simulink model "Parent"  (R2024a)
settings: Solver=FixedStepAuto  StartTime=0.0  StopTime=inf  RelTol=1e-3
libraries: androidcommunicationlib x3, androiduilib x3, androidaudiovideolib x2
settings Model: Creator=tamiz  LastModifiedBy=Shesh
settings OptimizationCC: EnhancedBackFolding=on  PassReuseOutputArgsAs=Individual arguments  ZeroExternalMemoryAtStartup=off  ZeroInternalMemoryAtStartup=off  MaxStackSize=64  OptimizeBlockOrder=speed  DifferentSizesBufferReuse=on  OptimizationCustomize=off  EfficientTunableParamExpr=on
settings DebuggingCC: ParameterTunabilityLossMsg=error
settings HardwareCC: ProdBitPerPointer=32  ProdBitPerSizeT=32  ProdBitPerPtrDiffT=32  ProdLargestAtomicInteger=Long  ProdLargestAtomicFloat=Double  ProdWordSize=32  ProdHWDeviceType=ARM Compatible->ARM Cortex  UseEmbeddedCoderFeatures=off  UseSimulinkCoderFeatures=off
settings SFSimCC: MATLABDynamicMemAlloc=off
settings RTWCC: Description=Embedded Coder  SystemTargetFile=ert.tlc  HardwareBoard=Android Device  TLCOptions="-aInlineSetEventsForThisBaseRateFcn=TLC_FALSE -aSuppressMultiTaskScheduler=TLC_FALSE  -aRateBasedStepFcn=0"  TemplateMakefile=ert_default_tmf  RTWVerbose=off  Toolchain=Android SDK/NDK Tools  GPUComputeCapability=3.5
settings CodeAppCC: ForceParamTrailComments=on  IgnoreCustomStorageClasses=off  OperatorAnnotations=on  SimulinkDataObjDesc=on  SFDataObjDesc=on  InsertBlockDesc=on
settings ERTTargetCC: SupportNonInlinedSFcns=on

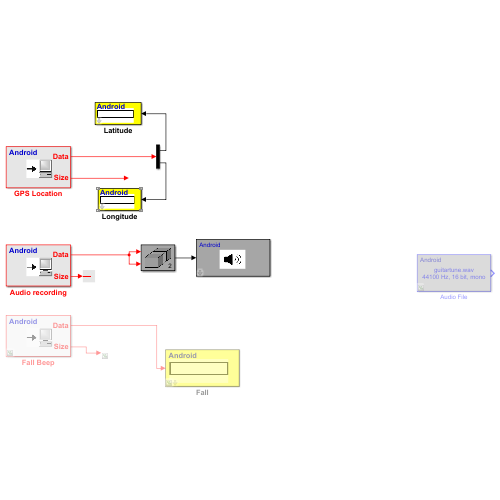
[thumbnail: Simulink's stored preview of the top-level diagram]
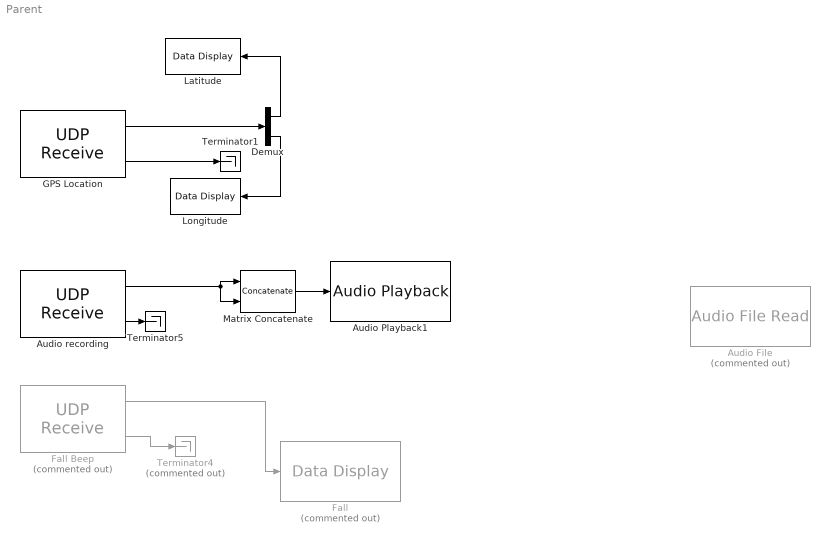
== system Parent ==
  Audio File : androidaudiovideolib/Audio File Read  Commented=on  FileName=C:\Users\tamiz\Downloads\beep-11.wav  FrameSize=4410
  Audio Playback1 : androidaudiovideolib/Audio Playback  SampleFreq=44100  AudioSamplingFreq=44100  SampleTime=0.1  DeviceStr=0  QueueDuration=0  BlockPlatform=Android
  Audio recording : androidcommunicationlib/UDP Receive  localURL='0.0.0.0'  localPort=25001  remoteURL='0.0.0.0'  remotePort=-1  recvBufferSize=8192  signalDatatype=int16  dims=4410  isVarSize=off  showBlockingTime=off  blockingTime=0  sampletime=0.1  blockPlatform=Android
  Demux : Demux  Outputs=2
  Fall : androiduilib/Data Display  Commented=on  DataDisplayId=Parent/Fall  Format=Integer  Precision=6  SimulateUsing=Code generation  blockPlatform=Android
  Fall Beep : androidcommunicationlib/UDP Receive  Commented=on  localURL='0.0.0.0'  localPort=25001  remoteURL='0.0.0.0'  remotePort=-1  recvBufferSize=8192  signalDatatype=int8  dims=1  isVarSize=off  showBlockingTime=off  blockingTime=0  sampletime=0.1  blockPlatform=Android
  GPS Location : androidcommunicationlib/UDP Receive  localURL='0.0.0.0'  localPort=25002  remoteURL='0.0.0.0'  remotePort=-1  recvBufferSize=8192  signalDatatype=double  dims=2  isVarSize=off  showBlockingTime=off  blockingTime=0  sampletime=0.1  blockPlatform=Android
  Latitude : androiduilib/Data Display  DataDisplayId=Parent/Latitude  Format=Float  Precision=10  SimulateUsing=Code generation  blockPlatform=Android
  Longitude : androiduilib/Data Display  DataDisplayId=Parent/Longitude  Format=Float  Precision=10  SimulateUsing=Code generation  blockPlatform=Android
  Matrix Concatenate : Concatenate  Mode=Multidimensional array  ConcatenateDimension=2
  Terminator1 : Terminator
  Terminator4 : Terminator  Commented=on
  Terminator5 : Terminator
  wires:
  GPS Location/2 -> Terminator1/1
  GPS Location/1 -> Demux/1
  Demux/1 -> Latitude/1
  Demux/2 -> Longitude/1
  Fall Beep/2 -> Terminator4/1
  Fall Beep/1 -> Fall/1
  Audio recording/2 -> Terminator5/1
  Matrix Concatenate/1 -> Audio Playback1/1
  Audio recording/1 -> Matrix Concatenate/2, Matrix Concatenate/1
